simulink model "Pv_array_three_phase_inverter"  (R2017b)
settings: Solver=VariableStepAuto  StartTime=0.0  StopTime=0.04  MaxStep=1e-4  RelTol=1e-3
libraries: powerlib x29, re_lib x1
settings Model: Creator=Ashish Kumar  LastModifiedBy=Ashish Kumar

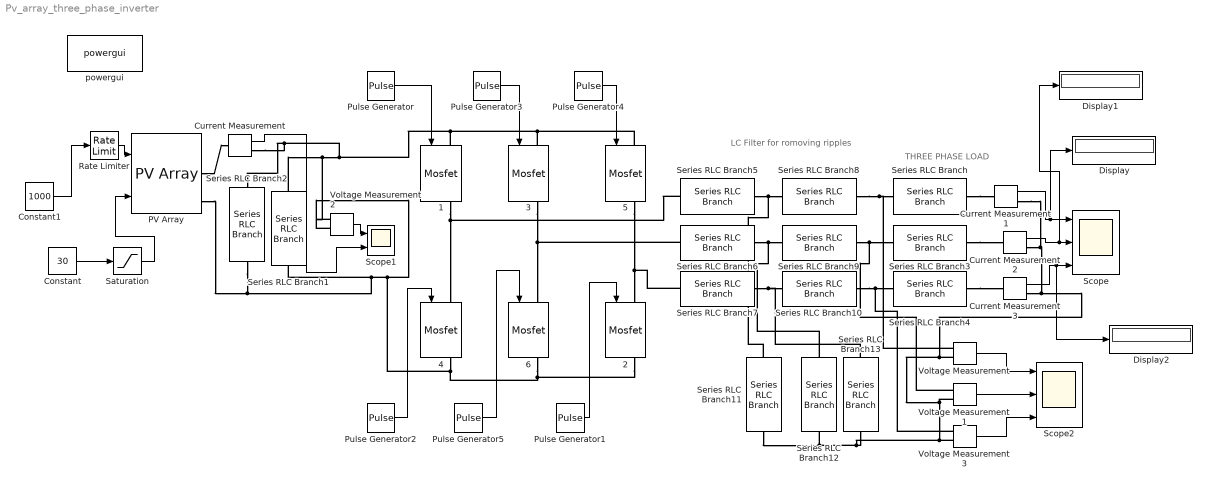
== system Pv_array_three_phase_inverter ==
  note: LC Filter for romoving ripples
  note: THREE PHASE LOAD
  {1..6} (6 alike) : powerlib/Power Electronics/Mosfet  Ron=0.1  Lon=0  Rd=0  Vfd=0  IC=0  Rs=1e5  Cs=inf  Measurements=on
  Constant : Constant  Value=30
  Constant1 : Constant  Value=1000
  Current Measurement{,1..3} (4 alike) : powerlib/Measurements/Current Measurement  PhasorSimulation=off  OutputType=Complex  PSBequivalent=0
  Display : Display
  Display1 : Display
  Display2 : Display
  PV Array : re_lib/Solar/PV Array  Npar=5  Nser=40  PlotType=array @ 1000 W/m2 & specified temperatures  S_vec="[ 1000  500  100 ]"  Temp_C_vec="[ 45 25  ]"  ModuleName=User-defined  PlotWhenSelected=off  Pm=243.412  Ncell=60  Voc=38.3  Isc=8.81  Vm=30.2  Im=8.06  beta_Voc_pc=-0.35601  alpha_Isc_pc=0.07  beta_Voc=-0.13635  alpha_Isc=0.006167  IL=8.8468  I0=2.613e-10  nI=1.0265  Rsh=103.8804  Rs=0.43387  BAL=off  Tc=1e-6  Tfilter=5e-5
  Pulse Generator : DiscretePulseGenerator  PulseType=Time based  Period=2e-3  PulseWidth=50
  Pulse Generator1 : DiscretePulseGenerator  PulseType=Time based  Period=2e-3  PulseWidth=50  PhaseDelay=2e-3/6
  Pulse Generator2 : DiscretePulseGenerator  PulseType=Time based  Period=2e-3  PulseWidth=50  PhaseDelay=2e-3/2
  Pulse Generator3 : DiscretePulseGenerator  PulseType=Time based  Period=2e-3  PulseWidth=50  PhaseDelay=2e-3/3
  Pulse Generator4 : DiscretePulseGenerator  PulseType=Time based  Period=2e-3  PulseWidth=50  PhaseDelay=2e-3*2/3
  Pulse Generator5 : DiscretePulseGenerator  PulseType=Time based  Period=2e-3  PulseWidth=50  PhaseDelay=2e-3*5/6
  Rate Limiter : RateLimiter  RisingSlewLimit=9000  FallingSlewLimit=-9000  SampleTimeMode=inherited  InitialCondition=1000
  Saturation : Saturate  UpperLimit=55  LowerLimit=25
  Scope : Scope  NumInputPorts=3
  Scope1 : Scope  NumInputPorts=2
  Scope2 : Scope  NumInputPorts=3
  Series RLC Branch : powerlib/Elements/Series RLC Branch  LConnTagsString=__new0  RConnTagsString=__new0  BranchType=RL  Resistance=10  Inductance=1e-3  SetiL0=off  InitialCurrent=0  Capacitance=1e-6  Setx0=off  InitialVoltage=0  Measurements=None
  Series RLC Branch1 : powerlib/Elements/Series RLC Branch  LConnTagsString=__new0  RConnTagsString=__new0  BranchType=R  Resistance=5  Inductance=1e-3  SetiL0=off  InitialCurrent=0  Capacitance=1e-6  Setx0=off  InitialVoltage=0  Measurements=None
  Series RLC Branch{5..10} (6 alike) : powerlib/Elements/Series RLC Branch  LConnTagsString=__new0  RConnTagsString=__new0  BranchType=L  Resistance=1  Inductance=0.01  SetiL0=off  InitialCurrent=0  Capacitance=1e-6  Setx0=off  InitialVoltage=0  Measurements=None
  Series RLC Branch11 : powerlib/Elements/Series RLC Branch  LConnTagsString=__new0  RConnTagsString=__new0  BranchType=C  Resistance=1  Inductance=1e-3  SetiL0=off  InitialCurrent=0  Capacitance=40e-6  Setx0=off  InitialVoltage=0  Measurements=None
  Series RLC Branch12 : powerlib/Elements/Series RLC Branch  LConnTagsString=__new0  RConnTagsString=__new0  BranchType=C  Resistance=1  Inductance=1e-3  SetiL0=off  InitialCurrent=0  Capacitance=40e-6  Setx0=off  InitialVoltage=0  Measurements=None
  Series RLC Branch13 : powerlib/Elements/Series RLC Branch  LConnTagsString=__new0  RConnTagsString=__new0  BranchType=C  Resistance=1  Inductance=1e-3  SetiL0=off  InitialCurrent=0  Capacitance=40e-6  Setx0=off  InitialVoltage=0  Measurements=None
  Series RLC Branch2 : powerlib/Elements/Series RLC Branch  LConnTagsString=__new0  RConnTagsString=__new0  BranchType=C  Resistance=1  Inductance=1e-3  SetiL0=off  InitialCurrent=0  Capacitance=1e-6  Setx0=off  InitialVoltage=0  Measurements=None
  Series RLC Branch3 : powerlib/Elements/Series RLC Branch  LConnTagsString=__new0  RConnTagsString=__new0  BranchType=RL  Resistance=10  Inductance=1e-3  SetiL0=off  InitialCurrent=0  Capacitance=1e-6  Setx0=off  InitialVoltage=0  Measurements=None
  Series RLC Branch4 : powerlib/Elements/Series RLC Branch  LConnTagsString=__new0  RConnTagsString=__new0  BranchType=RL  Resistance=10  Inductance=1e-3  SetiL0=off  InitialCurrent=0  Capacitance=1e-6  Setx0=off  InitialVoltage=0  Measurements=None
  Voltage Measurement{,1..3} (4 alike) : powerlib/Measurements/Voltage Measurement  PhasorSimulation=off  OutputType=Complex  PSBequivalent=0
  powergui : powerlib/powergui  Priority=1  SimulationMode=Continuous  SampleTime=50e-6  frequency=60  Iterations=50  frequencyindice=0  Pbase=100e6  ErrMax=1e-4  UnitsV=kV  UnitsW=MW  buscounter=0  FunctionMessages=off  echomessages=off  EnableUseOfTLC=off  CurrentSourceSwitches=off  DisableSnubberDevices=off  DisableRonSwitches=off  DisableVfSwitches=off  DisplayEquations=off  SolverType=Tustin/Backward Euler (TBE)  Interpol=off  ExternalGateDelay=off  methode=off  Ts=100  x0status=zero  SPID=on  SwTol=0  HookPort=off  RestoreLinks=warning  ResistiveCurrentMeasurement=off  Frange=[0:2:500]  Ylog=off  Xlog=on  ShowGrid=off  save=off  variable=ZData  structure=0  ZoomFFT=off  StartTime=0.0  cycles=1  DisplayStyle=1  fundamental=60  FreqAxis=off  MaxFrequency=1000  frequencyindicesteady=1  RmsSteady=1  display=off
  wires:
  Pulse Generator/1 -> 1/1
  Pulse Generator1/1 -> 2/1
  Pulse Generator2/1 -> 4/1
  Pulse Generator3/1 -> 3/1
  Pulse Generator4/1 -> 5/1
  Pulse Generator5/1 -> 6/1
  Saturation/1 -> PV Array/2
  Voltage Measurement2/1 -> Scope1/1
  Constant/1 -> Saturation/1
  Constant1/1 -> Rate Limiter/1
  Current Measurement/1 -> Scope1/2
  Rate Limiter/1 -> PV Array/1
  Current Measurement2/1 -> Display1/1, Scope/2
  Current Measurement1/1 -> Scope/1, Display/1
  Current Measurement3/1 -> Display2/1, Scope/3
  Voltage Measurement1/1 -> Scope2/2
  Voltage Measurement/1 -> Scope2/1
  Voltage Measurement3/1 -> Scope2/3
  connections:
  5/RConn1 -- Series RLC Branch7/LConn1 -- 2/LConn1
  3/RConn1 -- Series RLC Branch6/LConn1 -- 6/LConn1
  1/RConn1 -- Series RLC Branch5/LConn1 -- 4/LConn1
  PV Array/RConn2 -- Voltage Measurement2/LConn2 -- 2/RConn1 -- 6/RConn1 -- 4/RConn1 -- Series RLC Branch1/RConn1 -- Series RLC Branch2/RConn1
  Series RLC Branch1/LConn1 -- 5/LConn1 -- 3/LConn1 -- 1/LConn1 -- Series RLC Branch2/LConn1 -- Current Measurement/RConn1 -- Voltage Measurement2/LConn1
  PV Array/RConn1 -- Current Measurement/LConn1
  Series RLC Branch5/RConn1 -- Series RLC Branch11/LConn1 -- Series RLC Branch8/LConn1
  Series RLC Branch8/RConn1 -- Voltage Measurement/LConn1 -- Series RLC Branch/LConn1
  Series RLC Branch6/RConn1 -- Series RLC Branch12/LConn1 -- Series RLC Branch9/LConn1
  Series RLC Branch9/RConn1 -- Voltage Measurement1/LConn1 -- Series RLC Branch3/LConn1
  Series RLC Branch7/RConn1 -- Series RLC Branch13/LConn1 -- Series RLC Branch10/LConn1
  Series RLC Branch10/RConn1 -- Voltage Measurement3/LConn1 -- Series RLC Branch4/LConn1
  Series RLC Branch/RConn1 -- Current Measurement1/LConn1
  Series RLC Branch3/RConn1 -- Current Measurement2/LConn1
  Series RLC Branch4/RConn1 -- Current Measurement3/LConn1
  Series RLC Branch11/RConn1 -- Current Measurement1/RConn1 -- Current Measurement2/RConn1 -- Current Measurement3/RConn1 -- Voltage Measurement/LConn2 -- Voltage Measurement1/LConn2 -- Voltage Measurement3/LConn2 -- Series RLC Branch13/RConn1 -- Series RLC Branch12/RConn1
